simulink model "acc"  (R2025a)
settings: Solver=VariableStepAuto  StartTime=0.0  StopTime=10.0  RelTol=1e-3
settings Model: Creator=matthewkeller  LastModifiedBy=ryanjing

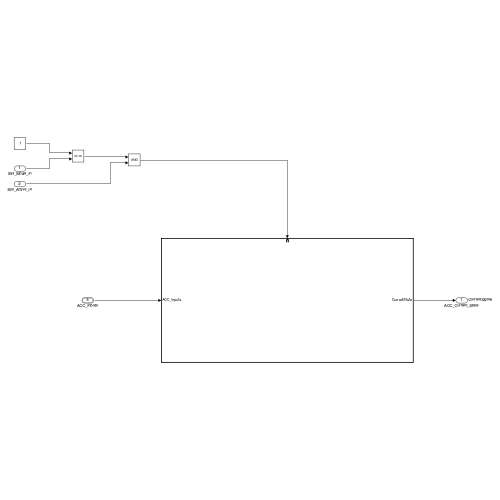
[thumbnail: Simulink's stored preview of the top-level diagram]
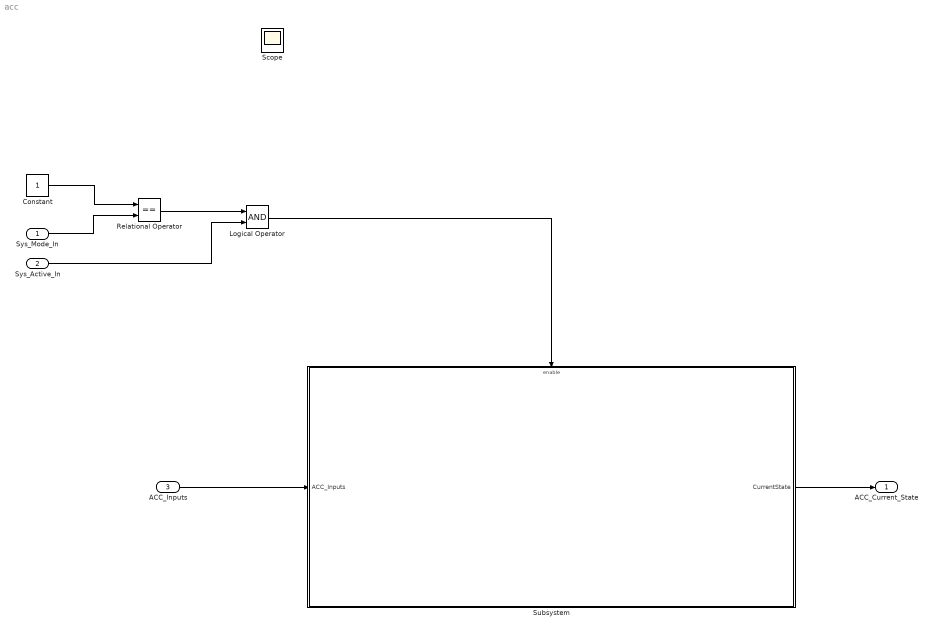
== system acc ==
  Sys_Mode_In : Inport  OutDataTypeStr=int8
  Sys_Active_In : Inport  Port=2  OutDataTypeStr=boolean
  ACC_Inputs : Inport  Port=3  OutDataTypeStr=Bus: ACCStatusBus
  Constant : Constant  OutDataTypeStr=int8
  Logical Operator : Logic  AllPortsSameDT=off  OutDataTypeStr=boolean
  Relational Operator : RelationalOperator  Operator===  OutDataTypeStr=boolean  RndMeth=Simplest  InputSameDT=off
  Subsystem : Subsystem
  ACC_Current_State : Outport  SignalName=CurrentSignal
  Scope : Scope
      settings: ActiveDisplayYMinimum=-1  ActiveDisplayYMaximum=1
  wires:
  Constant/1 -> Relational Operator/1
  Sys_Mode_In/1 -> Relational Operator/2
  Sys_Active_In/1 -> Logical Operator/2
  Relational Operator/1 -> Logical Operator/1
  Logical Operator/1 -> Subsystem/Enable
  ACC_Inputs/1 -> Subsystem/1(ACC_Inputs)
  Subsystem/1(CurrentState) -> ACC_Current_State/1

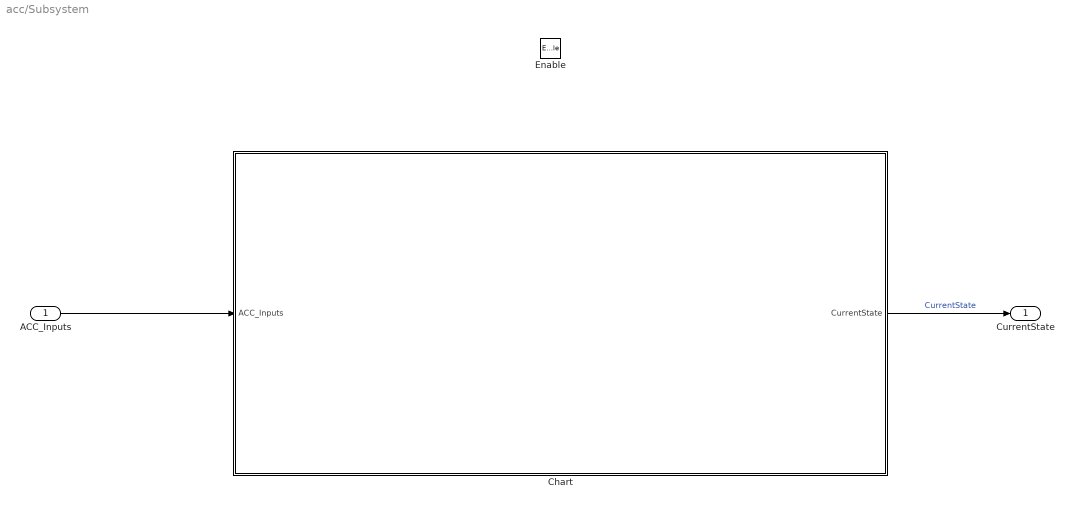
== system acc/Subsystem ==
  ACC_Inputs : Inport
  Enable : EnablePort
  Chart : Stateflow chart  TreatAsAtomicUnit=on
  CurrentState : Outport
  wires:
  Chart/1(CurrentState) -> CurrentState/1  "CurrentState"
  ACC_Inputs/1 -> Chart/1(ACC_Inputs)

== stateflow chart acc/Subsystem/Chart ==
  settings: executeAtInitialization=1
  state ACC_Deactivated
    entry:
    CurrentState = 0;
  state ACC_Active
    entry:
    CurrentState = 2;
  state ACC_Standby
    entry:
    CurrentState = 1;
  (default) -> ACC_Deactivated
  ACC_Active -> ACC_Deactivated [order 2] : [ACC_Inputs.Timeout_Event]
  ACC_Active -> ACC_Deactivated [order 1] : [ACC_Inputs.Cancel_Pressed || ACC_Inputs.Driver_Brakes]
  ACC_Deactivated -> ACC_Standby : [ACC_Inputs.ACC_Enable_Pressed && ACC_Inputs.V2X_Switch_ON && ACC_Inputs.Longitudinal_Switch_ON]
  ACC_Standby -> ACC_Active : [ACC_Inputs.Set_Resume && ACC_Inputs.In_CACC_Speed_Range]
  data: ACC_Inputs input Bus: ACCStatusBus; CurrentState output int8
